simulink model "rexus_project"  (R2025b)
settings: Solver=VariableStepAuto  StartTime=0.0  StopTime=10.0  RelTol=1e-3
values from neighbouring files (symbols this model uses):
  A = [10 2; 5 13]    [REXUS.m]
  B = [0 ; 0.1]    [REXUS.m]
  C = eye(2)    [REXUS.m]
  D = [0;0]    [REXUS.m]
settings Model: Creator=sofia  LastModifiedBy=sofia
settings SFSimCC: SimParseCustomCode=off  SimTargetLang=C++
settings SFSimCC: SimCustomHeaderCode=|
  | #include"solver_wrapper.hpp"
  | #include"qp_solver.hpp"
settings SFSimCC: SimUserSources=|
  | solver_wrapper.cpp
  | qp_solver.cpp
settings SFSimCC: SimUserIncludeDirs=|
  | /Users/sofia/Desktop/projects_4_exercise/simulink_projects
  | /opt/homebrew/opt/eigen/include/eigen3

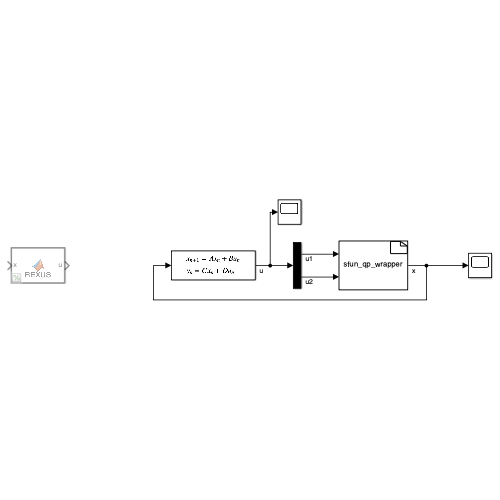
[thumbnail: Simulink's stored preview of the top-level diagram]
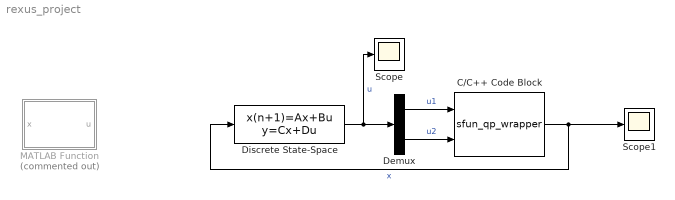
== system rexus_project ==
  C/C++ Code Block : S-Function  FunctionName=sfun_qp_wrapper  SFunctionDeploymentMode=off  EnableBusSupport=off  mask(S-Function Builder){}
      mask help: Simulink:masks:SFunctionBuilder_MD
      mask init:
      | val = [[.9  0.75 0.75 1 1 .9 .9 1]',[1 1 0.75 0.75 .9 .9 1 .9]'];try , sys = get_param(gcb,'SfunBuilderFcnName');if isempty(sys), sys = get_param(gcb,'FunctionName'); end,catch, sys = get_param(gcb,'FunctionName'); end
      settings: CopyFcn=set_param(gcbh,'LinkStatus','none')  OpenFcn=sfunctionwizard(gcbh)
      mask Display:
      | plot(val(:,1),val(:,2))
      | disp(sys)
  Demux : Demux  Outputs=2
  Discrete State-Space : DiscreteStateSpace  A=A  B=B  C=C  D=D  SampleTime=-1
  MATLAB Function : MATLAB Function  Commented=on  TreatAsAtomicUnit=on
  Scope : Scope
      settings: ActiveDisplayYMinimum=-1  ActiveDisplayYMaximum=1
  Scope1 : Scope
      settings: ActiveDisplayYMinimum=-1  ActiveDisplayYMaximum=1
  wires:
  Discrete State-Space/1 -> Scope/1, Demux/1  "u"
  Demux/1 -> C/C++ Code Block/1  "u1"
  Demux/2 -> C/C++ Code Block/2  "u2"
  C/C++ Code Block/1 -> Discrete State-Space/1, Scope1/1  "x"

== matlab function rexus_project/MATLAB Function ==
  data: x input; u output
function u = REXUS(x)
% REXUS CLF-QP controller (Simulink-compatible, no quadprog)
% x: 6x1 state vector
% u: 2x1 control output

% Ensure column vector
x = reshape(x,6,1);

% Default output
u = zeros(2,1);

% -------------------
% System parameters
J1  = 0.02;
J2  = 0.03;
Iw1 = 0.001;
Iw2 = 0.001;

% System matrices
A = [0 0 1 0 0 0;
     0 0 0 1 0 0;
     0 0 0 0 0 0;
     0 0 0 0 0 0;
     0 0 0 0 0 0;
     0 0 0 0 0 0];

B = [0 0;
     0 0;
    -1/J1 0;
     0 -1/J2;
     1/Iw1 0;
     0 1/Iw2];

% -------------------
% CLF parameters
P = diag([50 50 10 10 1 1]);
c = 2;

% Lyapunov terms
V   = x' * P * x;
LfV = 2 * x' * P * A * x;
LgV = 2 * x' * P * B;   % 1x2

% -------------------
% Manual CLF-QP solution (analytical)

% Nominal unconstrained control from Lyapunov derivative
u_nom = -LgV' * (V+c*V+LfV)/ (LgV*LgV');  

% Saturate control within bounds
u1 = min(max(u_nom(1), -0.2), 0.2);
u2 = min(max(u_nom(2), -0.2), 0.2);

u = [u1; u2];
